simulink model "scars_pwsat2_magne2"  (R2019b)
settings: Solver=ode14x  StartTime=0.0  StopTime=5*T  FixedStep=0.1  RelTol=1e-3
values from neighbouring files (symbols this model uses):
  initEuler = [0 0 0]    [SCARSSetup.m]    (also in pwsat2_setup.m; scars_setup.m)
undefined symbols (not defined in the file or in its folder): Earth, mag_sat, WGS84
libraries: scars_library x5, aerolibutil x3, sharedtransform x2, vrlib x1, aerolib6dof2 x1
settings Model: Creator=asmialek  LastModifiedBy=asmialek
settings DataIOCC: ReturnWorkspaceOutputsName=scars_out

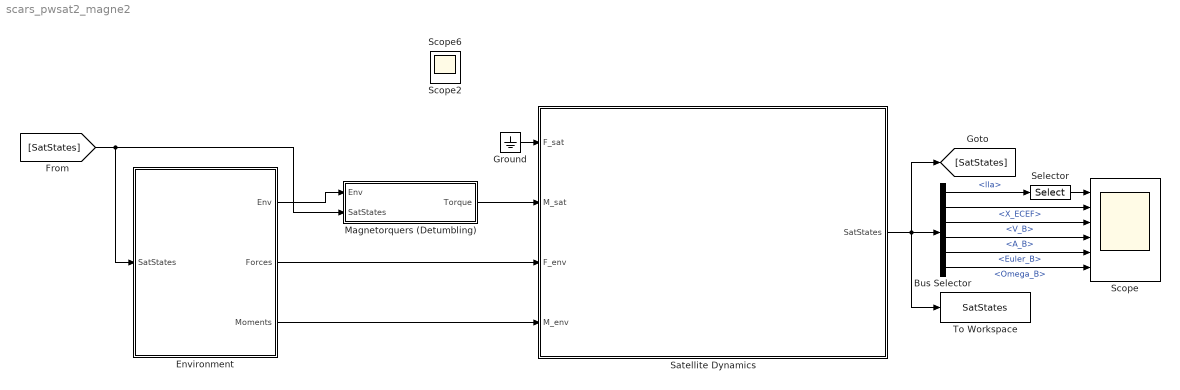
== system scars_pwsat2_magne2 ==
  Bus Selector : BusSelector  OutputSignals=lla,X_ECEF,V_B,A_B,Euler_B,Omega_B
  Environment : Subsystem  AncestorBlock=scars_library/Environment/Environment  mask{area_vector=[0 0 0]}
      mask prompts: area_vector "Area Vector"
  Ground : Ground
  Magnetorquers (Detumbling) : Subsystem  AncestorBlock=scars_library/Actuators/Magnetorquers (Detumbling)  mask(Magnetorquers){k_gain=-0.1, Parameter11=3, L_mt=2.666, R_mt=3.621, l_c_mt=0.25, w_c_mt=7.965e-3, d_w_mt=4.04e-4, mag_vol_max=5, Parameter9=0.2}
      mask prompts: k_gain "B-Dot algorithm gain"; Parameter11 "Maximum actuation error"; L_mt "Circuit inductance"; R_mt "Circuit resistance"; l_c_mt "Core length"; w_c_mt "Core width"; d_w_mt "Wire diameter"; mag_vol_max "Max voltage"; Parameter9 "Nominal magnetic dipole [Am^2]"
      mask help: A magnetorquer is an attitude actuator which uses Earth's geomagnetic field to generate controlling torque. The active part in the magnetorquer is the solenoid, which generates the magnetic dipole moment proportional to the current conducted by the coil.
      mask init:
      | gamma_mt = 2; % empirical constant
      | 
      | mt_pre = gamma_mt*pi*l_c_mt*w_c_mt/(4*d_w_mt);
      | mt_top = (((l_c_mt/w_c_mt)^2)-1)^(3/2);
      | mt_bottom = (l_c_mt/w_c_mt)*acosh(l_c_mt/w_c_mt)-sqrt((l_c_mt/w_c_mt)-1);
      | 
      | mt_gain = mt_pre*((mt_top/mt_bottom)-1);
  Satellite Dynamics : Subsystem  AncestorBlock=scars_library/Advanced/Satellite Dynamics
      mask Display: image('pw-sat-2__2.jpg'); % Use "Edit Image" on toolstrip to change.
  Scope : Scope  NumInputPorts=6
  Selector : Selector  InputPortWidth=3  IndexOptions=Index vector (dialog)  Indices=3  OutputSizes=1
  To Workspace : ToWorkspace  VariableName=SatStates  SaveFormat=Timeseries  SampleTime=-1
  Scope2 : Scope
  Scope6 : Scope
  wires:
  Bus Selector/2 -> Scope/2  "<X_ECEF>"
  Bus Selector/1 -> Selector/1  "<lla>"
  Selector/1 -> Scope/1
  Satellite Dynamics/1(SatStates) -> Bus Selector/1, [SatStates], To Workspace/1
  Bus Selector/3 -> Scope/3  "<V_B>"
  Bus Selector/4 -> Scope/4  "<A_B>"
  Bus Selector/5 -> Scope/5  "<Euler_B>"
  Bus Selector/6 -> Scope/6  "<Omega_B>"
  Environment/1(Env) -> Magnetorquers (Detumbling)/1(Env)
  [SatStates] -> Magnetorquers (Detumbling)/2(SatStates), Environment/1(SatStates)
  Environment/2(Forces) -> Satellite Dynamics/3(F_env)
  Environment/3(Moments) -> Satellite Dynamics/4(M_env)
  Magnetorquers (Detumbling)/1(Torque) -> Satellite Dynamics/2(M_sat)
  Ground/1 -> Satellite Dynamics/1(F_sat)

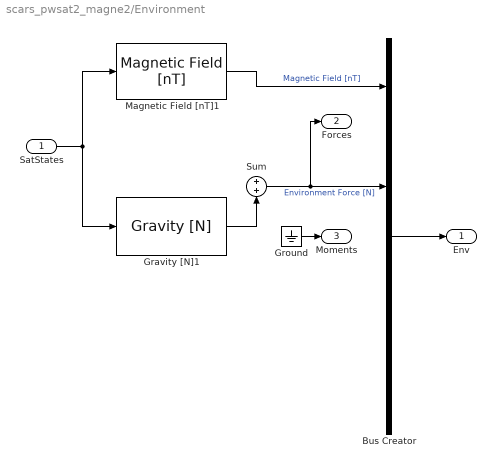
== system scars_pwsat2_magne2/Environment ==
  SatStates : Inport
  Bus Creator : BusCreator  Inputs=4
  Gravity [N]1 : scars_library/Environment/Gravity [N]  mass=1
  Ground : Ground
  Magnetic Field [nT]1 : scars_library/Environment/Magnetic Field [nT]  SystemSampleTime=-1  Latency=0  AutoFrameSizeCalculation=off
  Sum : Sum  Inputs=+|+
  Env : Outport
  Forces : Outport  Port=2
  Moments : Outport  Port=3
  wires:
  Ground/1 -> Moments/1
  Gravity [N]1/1 -> Sum/2
  Bus Creator/1 -> Env/1
  Magnetic Field [nT]1/1 -> Bus Creator/1  "Magnetic Field [nT]"
  Sum/1 -> Forces/1, Bus Creator/2  "Environment Force [N]"
  SatStates/1 -> Gravity [N]1/1, Magnetic Field [nT]1/1

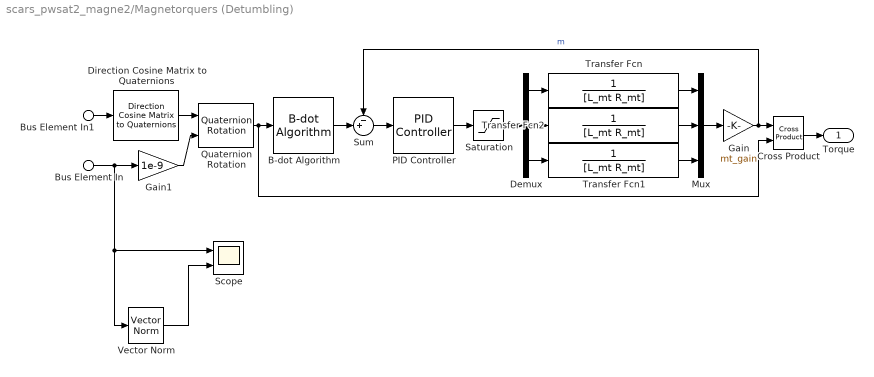
== system scars_pwsat2_magne2/Magnetorquers (Detumbling) ==
  Bus Element In : Inport  PortName=Env  Element=Magnetic Field [nT]
  Bus Element In1 : Inport  Port=2  PortName=SatStates  Element=DCM_NED2B
  B-dot Algorithm : scars_library/ Control Algorithms /B-dot Algorithm  k_gain=-0.1
  Cross Product : vrlib/Utilities/Cross Product
      settings: SourceProductName=Simulink
  Demux : Demux  Outputs=3
  Direction Cosine Matrix to Quaternions : sharedtransform/Direction Cosine Matrix  to Quaternions  aMode=0  action=None  tolerance=eps(2)
      settings: SourceProductName=Aerospace Blockset  SourceProductBaseCode=AE
  Gain : Gain  Gain=mt_gain
  Gain1 : Gain  Gain=1e-9
  Mux : Mux  Inputs=3
  PID Controller : scars_library/ Control Algorithms /PID Controller  Kp=1  Ki=0  Kd=0  pid_sat_max=inf  pid_sat_min=-inf  pid_dz_max=0  pid_dz_min=0
  Quaternion Rotation : aerolibutil/Quaternion Rotation
  Saturation : Saturate  UpperLimit=mag_sat  LowerLimit=-mag_sat
  Scope : Scope  NumInputPorts=2
  Sum : Sum  Inputs=-+|
  Transfer Fcn : TransferFcn  Denominator=[L_mt R_mt]
  Transfer Fcn1 : TransferFcn  Denominator=[L_mt R_mt]
  Transfer Fcn2 : TransferFcn  Denominator=[L_mt R_mt]
  Vector Norm : scars_library/Vector Norm  SystemSampleTime=-1  Latency=0  AutoFrameSizeCalculation=off
  Torque : Outport
  wires:
  Gain1/1 -> Quaternion Rotation/2
  Gain/1 -> Cross Product/1, Sum/1  "m"
  Bus Element In1/1 -> Direction Cosine Matrix to Quaternions/1
  Transfer Fcn2/1 -> Mux/2
  Cross Product/1 -> Torque/1
  Transfer Fcn1/1 -> Mux/3
  Bus Element In/1 -> Vector Norm/1, Scope/1, Gain1/1
  Transfer Fcn/1 -> Mux/1
  Demux/2 -> Transfer Fcn2/1
  Mux/1 -> Gain/1
  Quaternion Rotation/1 -> Cross Product/2, B-dot Algorithm/1
  Direction Cosine Matrix to Quaternions/1 -> Quaternion Rotation/1
  Sum/1 -> PID Controller/1
  Saturation/1 -> Demux/1
  Demux/1 -> Transfer Fcn/1
  B-dot Algorithm/1 -> Sum/2
  Demux/3 -> Transfer Fcn1/1
  PID Controller/1 -> Saturation/1
  Vector Norm/1 -> Scope/2

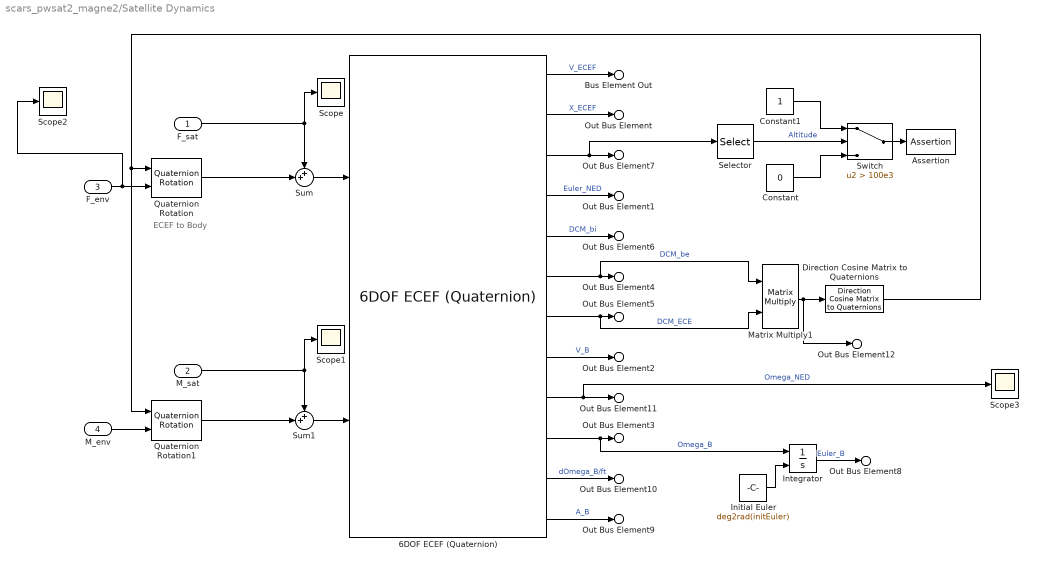
== system scars_pwsat2_magne2/Satellite Dynamics ==
  note: ECEF to Body
  F_sat : Inport
  M_sat : Inport  Port=2
  F_env : Inport  Port=3
  M_env : Inport  Port=4
  6DOF ECEF (Quaternion) : aerolib6dof2/6DOF ECEF (Quaternion)  units=Metric (MKS)  mtype=Fixed  xg_0=r_lla  Vm_0=v_b  eul_0=deg2rad(initEuler)  pm_0=[0.1 0.2 0.3]  mass_0=1  mass_e=0.5  mass_f=2.0  inertia=eye(3)  inertia_e=eye(3)  inertia_f=2*eye(3)  vre_flag=on  abi_flag=off  ptype=Earth (WGS84)  R=6378137  F=1/298.257223563  w_E=7292115e-11  angle_in=Internal  LG0=0  quat_statename=''  pm_statename=''  Vm_statename=''  posECEF_statename=''  posECI_statename=''  LG_statename=''  mass_statename=''
      settings: SourceProductName=Aerospace Blockset  SourceProductBaseCode=AE
  Assertion : Assertion
  Constant : Constant  Value=0
  Constant1 : Constant
  Direction Cosine Matrix to Quaternions : sharedtransform/Direction Cosine Matrix  to Quaternions  aMode=0  action=None  tolerance=eps(2)
      settings: SourceProductName=Aerospace Blockset  SourceProductBaseCode=AE
  Initial Euler : Constant  Value=deg2rad(initEuler)
  Integrator : Integrator  InitialConditionSource=external  WrapState=on
  Matrix Multiply1 : Product  Multiplication=Matrix(*)
  Quaternion Rotation : aerolibutil/Quaternion Rotation
  Quaternion Rotation1 : aerolibutil/Quaternion Rotation
  Scope{,1..3} (4 alike) : Scope
  Selector : Selector  InputPortWidth=3  IndexOptions=Index vector (dialog)  Indices=3  OutputSizes=1
  Sum : Sum  Inputs=++|
  Sum1 : Sum  Inputs=++|
  Switch : Switch  Criteria=u2 > Threshold  Threshold=100e3
  Bus Element Out : Outport  PortName=SatStates  Element=V_ECEF
  Out Bus Element : Outport  PortName=SatStates  Element=X_ECEF
  Out Bus Element1 : Outport  PortName=SatStates  Element=Euler_NED
  Out Bus Element2 : Outport  PortName=SatStates  Element=V_B
  Out Bus Element3 : Outport  PortName=SatStates  Element=Omega_B
  Out Bus Element6 : Outport  PortName=SatStates  Element=DCM_ECI2B
  Out Bus Element4 : Outport  PortName=SatStates  Element=DCM_NED2B
  Out Bus Element5 : Outport  PortName=SatStates  Element=DCM_ECEF2NED
  Out Bus Element7 : Outport  PortName=SatStates  Element=lla
  Out Bus Element8 : Outport  PortName=SatStates  Element=Euler_B
  Out Bus Element9 : Outport  PortName=SatStates  Element=A_B
  Out Bus Element10 : Outport  PortName=SatStates  Element=dOmega_B/dt
  Out Bus Element11 : Outport  PortName=SatStates  Element=Omega_NED
  Out Bus Element12 : Outport  PortName=SatStates  Element=DCM_ECEF2B
  wires:
  Constant/1 -> Switch/3
  6DOF ECEF (Quaternion)/9 -> Scope3/1, Out Bus Element11/1  "Omega_NED"
  Initial Euler/1 -> Integrator/2
  M_env/1 -> Quaternion Rotation1/2
  6DOF ECEF (Quaternion)/12 -> Out Bus Element9/1  "A_B"
  6DOF ECEF (Quaternion)/7 -> Matrix Multiply1/2, Out Bus Element5/1  "DCM_ECE"
  6DOF ECEF (Quaternion)/11 -> Out Bus Element10/1  "dOmega_B/ft"
  6DOF ECEF (Quaternion)/3 -> Selector/1, Out Bus Element7/1
  6DOF ECEF (Quaternion)/5 -> Out Bus Element6/1  "DCM_bi"
  Sum/1 -> 6DOF ECEF (Quaternion)/1
  Integrator/1 -> Out Bus Element8/1  "Euler_B"
  Direction Cosine Matrix to Quaternions/1 -> Quaternion Rotation1/1, Quaternion Rotation/1
  F_sat/1 -> Scope/1, Sum/1
  Quaternion Rotation/1 -> Sum/2
  Quaternion Rotation1/1 -> Sum1/2
  Sum1/1 -> 6DOF ECEF (Quaternion)/2
  Matrix Multiply1/1 -> Direction Cosine Matrix to Quaternions/1, Out Bus Element12/1
  6DOF ECEF (Quaternion)/1 -> Bus Element Out/1  "V_ECEF"
  Selector/1 -> Switch/2  "Altitude"
  6DOF ECEF (Quaternion)/4 -> Out Bus Element1/1  "Euler_NED"
  6DOF ECEF (Quaternion)/6 -> Matrix Multiply1/1, Out Bus Element4/1  "DCM_be"
  6DOF ECEF (Quaternion)/2 -> Out Bus Element/1  "X_ECEF"
  Switch/1 -> Assertion/1
  Constant1/1 -> Switch/1
  6DOF ECEF (Quaternion)/10 -> Integrator/1, Out Bus Element3/1  "Omega_B"
  6DOF ECEF (Quaternion)/8 -> Out Bus Element2/1  "V_B"
  M_sat/1 -> Sum1/1, Scope1/1
  F_env/1 -> Scope2/1, Quaternion Rotation/2
